simulink library "Bit_Demultiplexers_Lib"  (Simulink 8.7)
settings: Solver=ode45  StartTime=0.0  StopTime=10.0  RelTol=1e-3
libraries: Bit_Demultiplexers_Lib x17
settings Model: Creator=uzivatel  LastModifiedBy=Jozko Mrkvicka

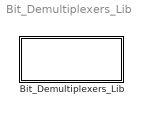
== system Bit_Demultiplexers_Lib ==
  Bit_Demultiplexers_Lib : Subsystem

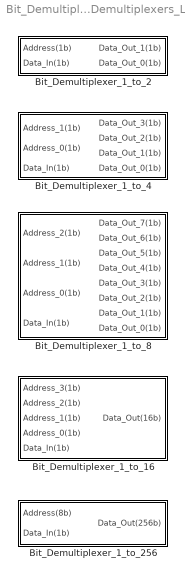
== system Bit_Demultiplexers_Lib/Bit_Demultiplexers_Lib ==
  Bit_Demultiplexer_1_to_16 : Subsystem
  Bit_Demultiplexer_1_to_2 : Subsystem
  Bit_Demultiplexer_1_to_256 : Subsystem
  Bit_Demultiplexer_1_to_4 : Subsystem
  Bit_Demultiplexer_1_to_8 : Subsystem

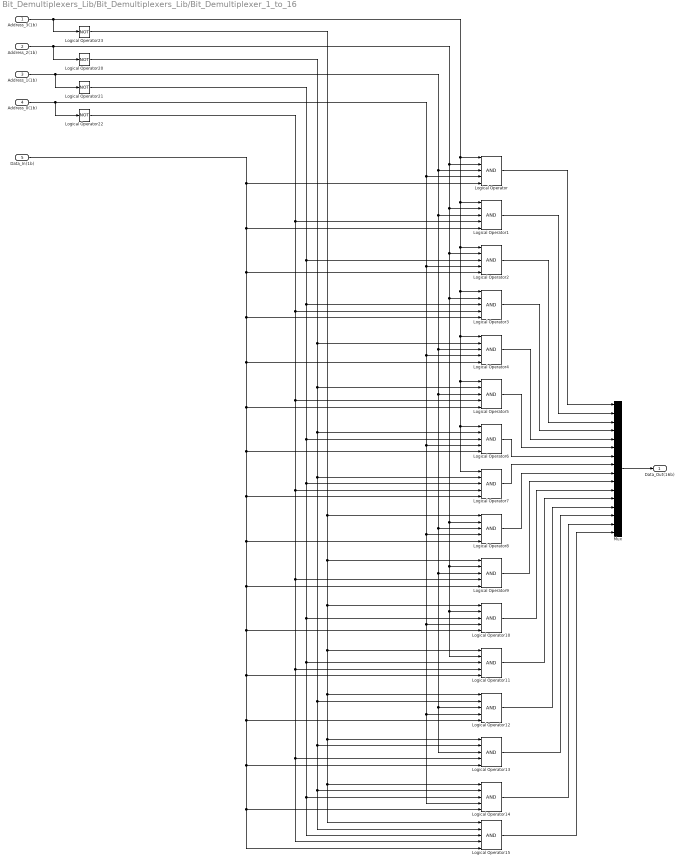
== system Bit_Demultiplexers_Lib/Bit_Demultiplexers_Lib/Bit_Demultiplexer_1_to_16 ==
  Address_3(1b) : Inport
  Address_2(1b) : Inport  Port=2
  Address_1(1b) : Inport  Port=3
  Address_0(1b) : Inport  Port=4
  Data_In(1b) : Inport  Port=5
  Logical Operator{,1..15} (16 alike) : Logic  Inputs=5  IconShape=distinctive  AllPortsSameDT=off  OutDataTypeStr=boolean
  Logical Operator{20..23} (4 alike) : Logic  Operator=NOT  Inputs=4  IconShape=distinctive  AllPortsSameDT=off  OutDataTypeStr=boolean
  Mux : Mux  Inputs=16
  Data_Out(16b) : Outport
  wires:
  Mux/1 -> Data_Out(16b)/1
  Logical Operator22/1 -> Logical Operator15/4, Logical Operator13/4, Logical Operator11/4, Logical Operator9/4, Logical Operator7/4, Logical Operator5/4, Logical Operator3/4, Logical Operator1/4
  Address_0(1b)/1 -> Logical Operator14/4, Logical Operator12/4, Logical Operator10/4, Logical Operator8/4, Logical Operator6/4, Logical Operator4/4, Logical Operator2/4, Logical Operator/4, Logical Operator22/1
  Logical Operator21/1 -> Logical Operator15/3, Logical Operator14/3, Logical Operator11/3, Logical Operator10/3, Logical Operator7/3, Logical Operator6/3, Logical Operator3/3, Logical Operator2/3
  Address_1(1b)/1 -> Logical Operator13/3, Logical Operator12/3, Logical Operator9/3, Logical Operator8/3, Logical Operator5/3, Logical Operator4/3, Logical Operator1/3, Logical Operator/3, Logical Operator21/1
  Logical Operator20/1 -> Logical Operator15/2, Logical Operator14/2, Logical Operator13/2, Logical Operator12/2, Logical Operator7/2, Logical Operator6/2, Logical Operator5/2, Logical Operator4/2
  Address_2(1b)/1 -> Logical Operator11/2, Logical Operator10/2, Logical Operator9/2, Logical Operator8/2, Logical Operator3/2, Logical Operator2/2, Logical Operator1/2, Logical Operator/2, Logical Operator20/1
  Logical Operator23/1 -> Logical Operator15/1, Logical Operator14/1, Logical Operator13/1, Logical Operator12/1, Logical Operator11/1, Logical Operator10/1, Logical Operator9/1, Logical Operator8/1
  Address_3(1b)/1 -> Logical Operator7/1, Logical Operator6/1, Logical Operator5/1, Logical Operator4/1, Logical Operator3/1, Logical Operator2/1, Logical Operator1/1, Logical Operator/1, Logical Operator23/1
  Data_In(1b)/1 -> Logical Operator/5, Logical Operator3/5, Logical Operator7/5, Logical Operator8/5, Logical Operator9/5, Logical Operator10/5, Logical Operator11/5, Logical Operator15/5, Logical Operator14/5, Logical Operator13/5, Logical Operator12/5, Logical Operator6/5, Logical Operator5/5, Logical Operator4/5, Logical Operator2/5, Logical Operator1/5
  Logical Operator15/1 -> Mux/16
  Logical Operator14/1 -> Mux/15
  Logical Operator13/1 -> Mux/14
  Logical Operator/1 -> Mux/1
  Logical Operator1/1 -> Mux/2
  Logical Operator2/1 -> Mux/3
  Logical Operator3/1 -> Mux/4
  Logical Operator4/1 -> Mux/5
  Logical Operator12/1 -> Mux/13
  Logical Operator11/1 -> Mux/12
  Logical Operator5/1 -> Mux/6
  Logical Operator10/1 -> Mux/11
  Logical Operator9/1 -> Mux/10
  Logical Operator6/1 -> Mux/7
  Logical Operator8/1 -> Mux/9
  Logical Operator7/1 -> Mux/8

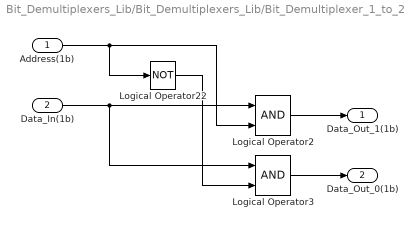
== system Bit_Demultiplexers_Lib/Bit_Demultiplexers_Lib/Bit_Demultiplexer_1_to_2 ==
  Address(1b) : Inport
  Data_In(1b) : Inport  Port=2
  Logical Operator2 : Logic  IconShape=distinctive  AllPortsSameDT=off  OutDataTypeStr=boolean
  Logical Operator22 : Logic  Operator=NOT  Inputs=4  IconShape=distinctive  AllPortsSameDT=off  OutDataTypeStr=boolean
  Logical Operator3 : Logic  IconShape=distinctive  AllPortsSameDT=off  OutDataTypeStr=boolean
  Data_Out_1(1b) : Outport
  Data_Out_0(1b) : Outport  Port=2
  wires:
  Logical Operator3/1 -> Data_Out_0(1b)/1
  Logical Operator2/1 -> Data_Out_1(1b)/1
  Logical Operator22/1 -> Logical Operator3/2
  Address(1b)/1 -> Logical Operator2/2, Logical Operator22/1
  Data_In(1b)/1 -> Logical Operator2/1, Logical Operator3/1

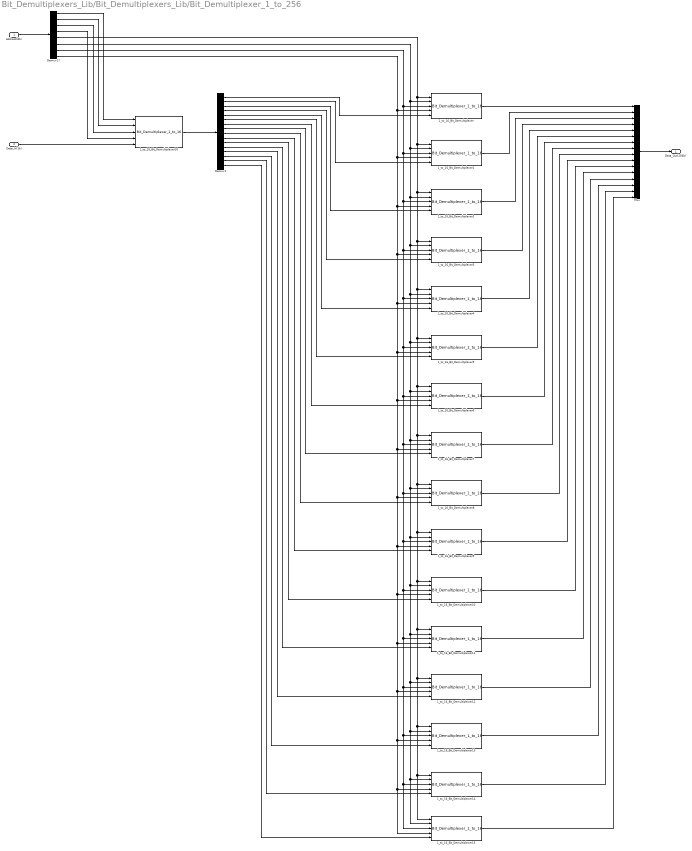
== system Bit_Demultiplexers_Lib/Bit_Demultiplexers_Lib/Bit_Demultiplexer_1_to_256 ==
  Address(8b) : Inport
  Data_In(1b) : Inport  Port=2
  1_to_16_Bit_Demultiplexer{,1..16} (17 alike) : Bit_Demultiplexers_Lib/Bit_Demultiplexers_Lib/Bit_Demultiplexer_1_to_16
  Demux1 : Demux  Outputs=16
  Demux17 : Demux  Outputs=8
  Mux : Mux  Inputs=16
  Data_Out(256b) : Outport  OutDataTypeStr=boolean
  wires:
  Mux/1 -> Data_Out(256b)/1
  Demux17/4 -> 1_to_16_Bit_Demultiplexer16/4
  Demux17/3 -> 1_to_16_Bit_Demultiplexer16/3
  Demux17/2 -> 1_to_16_Bit_Demultiplexer16/2
  Demux17/1 -> 1_to_16_Bit_Demultiplexer16/1
  Demux1/16 -> 1_to_16_Bit_Demultiplexer15/5
  Demux1/15 -> 1_to_16_Bit_Demultiplexer14/5
  Demux1/14 -> 1_to_16_Bit_Demultiplexer13/5
  Demux1/13 -> 1_to_16_Bit_Demultiplexer12/5
  Demux1/12 -> 1_to_16_Bit_Demultiplexer11/5
  Demux1/11 -> 1_to_16_Bit_Demultiplexer10/5
  Demux1/10 -> 1_to_16_Bit_Demultiplexer9/5
  Demux1/9 -> 1_to_16_Bit_Demultiplexer8/5
  Demux1/8 -> 1_to_16_Bit_Demultiplexer7/5
  Demux1/7 -> 1_to_16_Bit_Demultiplexer6/5
  Demux1/6 -> 1_to_16_Bit_Demultiplexer5/5
  Demux1/5 -> 1_to_16_Bit_Demultiplexer4/5
  Demux1/4 -> 1_to_16_Bit_Demultiplexer3/5
  Demux1/3 -> 1_to_16_Bit_Demultiplexer2/5
  Demux1/2 -> 1_to_16_Bit_Demultiplexer1/5
  Demux1/1 -> 1_to_16_Bit_Demultiplexer/5
  1_to_16_Bit_Demultiplexer16/1 -> Demux1/1
  Data_In(1b)/1 -> 1_to_16_Bit_Demultiplexer16/5
  1_to_16_Bit_Demultiplexer/1 -> Mux/1
  1_to_16_Bit_Demultiplexer1/1 -> Mux/2
  1_to_16_Bit_Demultiplexer2/1 -> Mux/3
  1_to_16_Bit_Demultiplexer3/1 -> Mux/4
  1_to_16_Bit_Demultiplexer15/1 -> Mux/16
  1_to_16_Bit_Demultiplexer14/1 -> Mux/15
  1_to_16_Bit_Demultiplexer13/1 -> Mux/14
  1_to_16_Bit_Demultiplexer12/1 -> Mux/13
  1_to_16_Bit_Demultiplexer11/1 -> Mux/12
  1_to_16_Bit_Demultiplexer10/1 -> Mux/11
  1_to_16_Bit_Demultiplexer9/1 -> Mux/10
  1_to_16_Bit_Demultiplexer8/1 -> Mux/9
  1_to_16_Bit_Demultiplexer7/1 -> Mux/8
  1_to_16_Bit_Demultiplexer6/1 -> Mux/7
  1_to_16_Bit_Demultiplexer5/1 -> Mux/6
  1_to_16_Bit_Demultiplexer4/1 -> Mux/5
  Demux17/5 -> 1_to_16_Bit_Demultiplexer/1, 1_to_16_Bit_Demultiplexer1/1, 1_to_16_Bit_Demultiplexer2/1, 1_to_16_Bit_Demultiplexer3/1, 1_to_16_Bit_Demultiplexer4/1, 1_to_16_Bit_Demultiplexer5/1, 1_to_16_Bit_Demultiplexer6/1, 1_to_16_Bit_Demultiplexer7/1, 1_to_16_Bit_Demultiplexer8/1, 1_to_16_Bit_Demultiplexer9/1, 1_to_16_Bit_Demultiplexer10/1, 1_to_16_Bit_Demultiplexer11/1, 1_to_16_Bit_Demultiplexer12/1, 1_to_16_Bit_Demultiplexer13/1, 1_to_16_Bit_Demultiplexer14/1, 1_to_16_Bit_Demultiplexer15/1
  Address(8b)/1 -> Demux17/1
  Demux17/7 -> 1_to_16_Bit_Demultiplexer/3, 1_to_16_Bit_Demultiplexer1/3, 1_to_16_Bit_Demultiplexer2/3, 1_to_16_Bit_Demultiplexer3/3, 1_to_16_Bit_Demultiplexer4/3, 1_to_16_Bit_Demultiplexer5/3, 1_to_16_Bit_Demultiplexer6/3, 1_to_16_Bit_Demultiplexer7/3, 1_to_16_Bit_Demultiplexer8/3, 1_to_16_Bit_Demultiplexer9/3, 1_to_16_Bit_Demultiplexer10/3, 1_to_16_Bit_Demultiplexer11/3, 1_to_16_Bit_Demultiplexer12/3, 1_to_16_Bit_Demultiplexer13/3, 1_to_16_Bit_Demultiplexer14/3, 1_to_16_Bit_Demultiplexer15/3
  Demux17/6 -> 1_to_16_Bit_Demultiplexer/2, 1_to_16_Bit_Demultiplexer1/2, 1_to_16_Bit_Demultiplexer2/2, 1_to_16_Bit_Demultiplexer3/2, 1_to_16_Bit_Demultiplexer4/2, 1_to_16_Bit_Demultiplexer5/2, 1_to_16_Bit_Demultiplexer6/2, 1_to_16_Bit_Demultiplexer7/2, 1_to_16_Bit_Demultiplexer8/2, 1_to_16_Bit_Demultiplexer9/2, 1_to_16_Bit_Demultiplexer10/2, 1_to_16_Bit_Demultiplexer11/2, 1_to_16_Bit_Demultiplexer12/2, 1_to_16_Bit_Demultiplexer13/2, 1_to_16_Bit_Demultiplexer14/2, 1_to_16_Bit_Demultiplexer15/2
  Demux17/8 -> 1_to_16_Bit_Demultiplexer/4, 1_to_16_Bit_Demultiplexer1/4, 1_to_16_Bit_Demultiplexer2/4, 1_to_16_Bit_Demultiplexer3/4, 1_to_16_Bit_Demultiplexer4/4, 1_to_16_Bit_Demultiplexer5/4, 1_to_16_Bit_Demultiplexer6/4, 1_to_16_Bit_Demultiplexer7/4, 1_to_16_Bit_Demultiplexer8/4, 1_to_16_Bit_Demultiplexer9/4, 1_to_16_Bit_Demultiplexer10/4, 1_to_16_Bit_Demultiplexer11/4, 1_to_16_Bit_Demultiplexer12/4, 1_to_16_Bit_Demultiplexer13/4, 1_to_16_Bit_Demultiplexer14/4, 1_to_16_Bit_Demultiplexer15/4

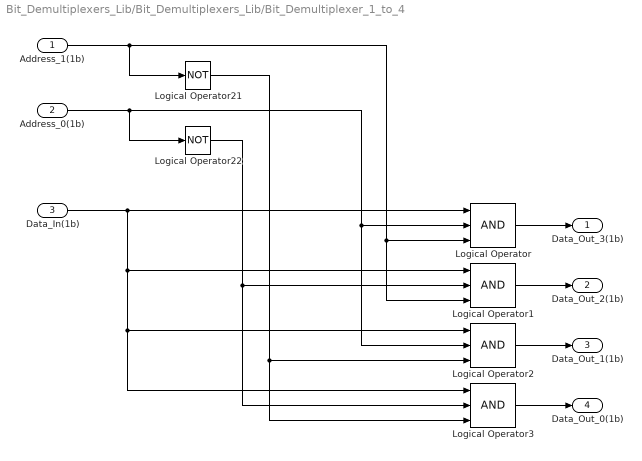
== system Bit_Demultiplexers_Lib/Bit_Demultiplexers_Lib/Bit_Demultiplexer_1_to_4 ==
  Address_1(1b) : Inport
  Address_0(1b) : Inport  Port=2
  Data_In(1b) : Inport  Port=3
  Logical Operator{,1..3} (4 alike) : Logic  Inputs=3  IconShape=distinctive  AllPortsSameDT=off  OutDataTypeStr=boolean
  Logical Operator21 : Logic  Operator=NOT  Inputs=4  IconShape=distinctive  AllPortsSameDT=off  OutDataTypeStr=boolean
  Logical Operator22 : Logic  Operator=NOT  Inputs=4  IconShape=distinctive  AllPortsSameDT=off  OutDataTypeStr=boolean
  Data_Out_3(1b) : Outport
  Data_Out_2(1b) : Outport  Port=2
  Data_Out_1(1b) : Outport  Port=3
  Data_Out_0(1b) : Outport  Port=4
  wires:
  Logical Operator3/1 -> Data_Out_0(1b)/1
  Logical Operator2/1 -> Data_Out_1(1b)/1
  Logical Operator1/1 -> Data_Out_2(1b)/1
  Logical Operator/1 -> Data_Out_3(1b)/1
  Logical Operator22/1 -> Logical Operator1/2, Logical Operator3/2
  Address_0(1b)/1 -> Logical Operator2/2, Logical Operator/2, Logical Operator22/1
  Logical Operator21/1 -> Logical Operator2/3, Logical Operator3/3
  Address_1(1b)/1 -> Logical Operator1/3, Logical Operator/3, Logical Operator21/1
  Data_In(1b)/1 -> Logical Operator/1, Logical Operator1/1, Logical Operator2/1, Logical Operator3/1

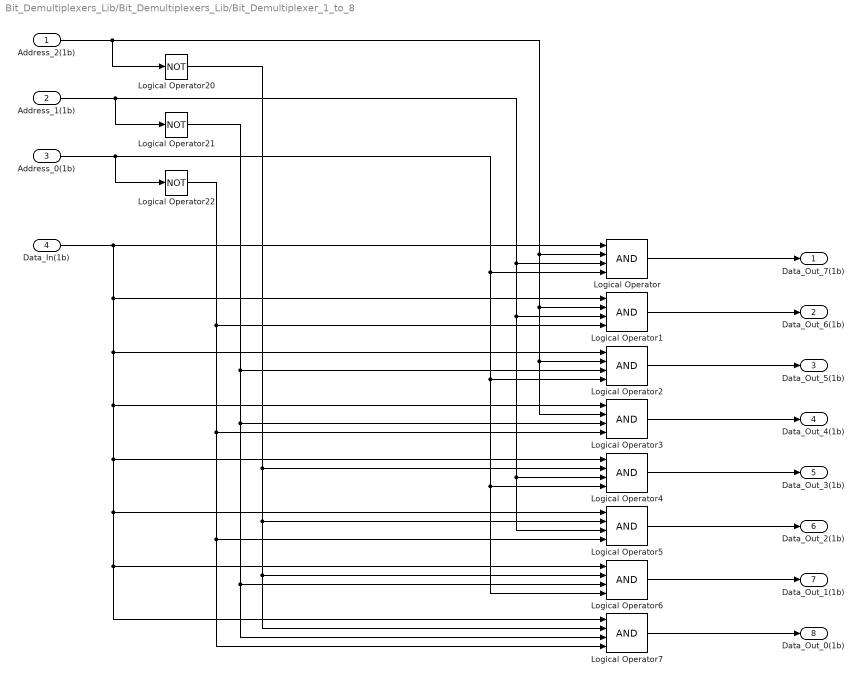
== system Bit_Demultiplexers_Lib/Bit_Demultiplexers_Lib/Bit_Demultiplexer_1_to_8 ==
  Address_2(1b) : Inport
  Address_1(1b) : Inport  Port=2
  Address_0(1b) : Inport  Port=3
  Data_In(1b) : Inport  Port=4
  Logical Operator{,1..7} (8 alike) : Logic  Inputs=4  IconShape=distinctive  AllPortsSameDT=off  OutDataTypeStr=boolean
  Logical Operator20 : Logic  Operator=NOT  Inputs=4  IconShape=distinctive  AllPortsSameDT=off  OutDataTypeStr=boolean
  Logical Operator21 : Logic  Operator=NOT  Inputs=4  IconShape=distinctive  AllPortsSameDT=off  OutDataTypeStr=boolean
  Logical Operator22 : Logic  Operator=NOT  Inputs=4  IconShape=distinctive  AllPortsSameDT=off  OutDataTypeStr=boolean
  Data_Out_7(1b) : Outport
  Data_Out_6(1b) : Outport  Port=2
  Data_Out_5(1b) : Outport  Port=3
  Data_Out_4(1b) : Outport  Port=4
  Data_Out_3(1b) : Outport  Port=5
  Data_Out_2(1b) : Outport  Port=6
  Data_Out_1(1b) : Outport  Port=7
  Data_Out_0(1b) : Outport  Port=8
  wires:
  Logical Operator6/1 -> Data_Out_1(1b)/1
  Logical Operator5/1 -> Data_Out_2(1b)/1
  Logical Operator4/1 -> Data_Out_3(1b)/1
  Logical Operator3/1 -> Data_Out_4(1b)/1
  Logical Operator2/1 -> Data_Out_5(1b)/1
  Logical Operator1/1 -> Data_Out_6(1b)/1
  Logical Operator/1 -> Data_Out_7(1b)/1
  Logical Operator22/1 -> Logical Operator1/4, Logical Operator3/4, Logical Operator5/4, Logical Operator7/4
  Address_0(1b)/1 -> Logical Operator2/4, Logical Operator4/4, Logical Operator6/4, Logical Operator/4, Logical Operator22/1
  Logical Operator21/1 -> Logical Operator2/3, Logical Operator3/3, Logical Operator6/3, Logical Operator7/3
  Address_1(1b)/1 -> Logical Operator1/3, Logical Operator4/3, Logical Operator5/3, Logical Operator/3, Logical Operator21/1
  Logical Operator20/1 -> Logical Operator4/2, Logical Operator5/2, Logical Operator6/2, Logical Operator7/2
  Address_2(1b)/1 -> Logical Operator1/2, Logical Operator2/2, Logical Operator3/2, Logical Operator/2, Logical Operator20/1
  Data_In(1b)/1 -> Logical Operator/1, Logical Operator1/1, Logical Operator2/1, Logical Operator3/1, Logical Operator4/1, Logical Operator5/1, Logical Operator6/1, Logical Operator7/1
  Logical Operator7/1 -> Data_Out_0(1b)/1
